simulink model "WebcamTester3"  (Simulink 7.3)
settings: Solver=FixedStepDiscrete  StartTime=0.0  StopTime=inf  MaxStep=0.2  RelTol=1e-3
settings Model: Creator=gclayton  LastModifiedBy=wildcat
settings DebuggingCC: InheritedTsInSrcMsg=none
settings RTWCC: SystemTargetFile=rlnx.tlc  GenCodeOnly=on  TemplateMakefile=rlnx_ubuntu.tmf  Description=Linux Real-Time Target  ProcessScript=rlnx_make_rtw_hook
settings RTWCC: CustomInclude=|
  | /usr/local/include/opencv/
  | /usr/local/include/
settings CodeAppCC: GenerateComments=off  SimulinkBlockComments=off
settings STFCustomTargetCC: ModelReferenceCompliant=off  MatFileLogging=on  SystemTargetFile=rlnx.tlc
settings GRTTargetCC: ModelReferenceCompliant=off  ParMdlRefBuildCompliant=off  CompOptLevelCompliant=off
settings CustomProperty: DataType=string  Value=-lm -ldl /usr/local/lib/libopencv_highgui.so.2.4 /usr/local/lib/libopencv_core.so.2.4 /usr/local/lib/libopencv_imgproc.so.2.4
settings EnumStrPairs: String=PC

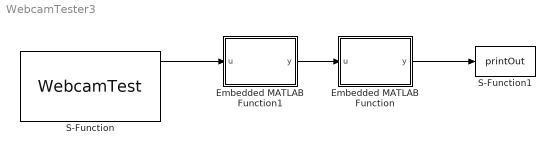
== system WebcamTester3 ==
  Embedded MATLAB Function : Stateflow chart  TreatAsAtomicUnit=on
  Embedded MATLAB Function1 : Stateflow chart  TreatAsAtomicUnit=on
  S-Function : S-Function  FunctionName=WebcamTest  EnableBusSupport=off
  S-Function1 : S-Function  FunctionName=printOut  EnableBusSupport=off
  wires:
  S-Function/1 -> Embedded MATLAB Function1/1(u)
  Embedded MATLAB Function/1(y) -> S-Function1/1
  Embedded MATLAB Function1/1(y) -> Embedded MATLAB Function/1(u)

== matlab function Embedded MATLAB Function1 ==
  data: u input double; y output double
function y = fcn(u)

y = uint32(u);

== matlab function Embedded MATLAB Function ==
  data: u input double; y output double
function y = fcn(u)

y = u(100,100);
